simulink model "power_PVarray_3500W"  (R2024b)
settings: Solver=FixedStepDiscrete  StartTime=0.0  StopTime=1.2  RelTol=1e-3
PreLoadFcn:
  | %
  | Fc=3780;                          % PWM Carrier frequency (Hz)
  | Ts_Power=1/Fc/200;         % Simscape Power Systems sample time (s)
  | Ts_Control=20*Ts_Power;  % Inverter Control system sample time (s)
InitFcn:
  | %
  | Fc=3780;                          % PWM Carrier frequency (Hz)
  | Ts_Power=1/Fc/200;         % Simscape Power Systems sample time (s)
  | Ts_Control=20*Ts_Power;  % Inverter Control system sample time (s)
libraries: spsSeriesRLCBranchLib x8, spsGroundLib x4, spsVoltageMeasurementLib x3, spsMeanLib x3, spsCurrentMeasurementLib x2, slpidlib x2, spsParallelRLCLoadLib x2, spsLinearTransformerLib x1, spsSeriesRLCLoadLib x1, spsUniversalBridgeLib x1, spsFundamentalPLLDrivenLib x1, spsPLLLib x1
Description:
  | Copyright 2008-2017 The MathWorks, Inc.
settings Model: Creator=MathWorks  LastModifiedBy=Lenovo
settings SolverCC: AlgebraicLoopSolver=TrustRegion
settings DataIOCC: SaveFormat=Structure  SignalLoggingSaveFormat=ModelDataLogs  SaveOutput=off  SignalLogging=off  DSMLogging=off  SaveTime=off  ReturnWorkspaceOutputs=off
settings OptimizationCC: ExpressionDepthLimit=2147483647  LifeSpan=inf
settings DebuggingCC: UnderspecifiedInitializationDetection=Classic  MergeDetectMultiDrivingBlocksExec=none  SolverPrmCheckMsg=warning  FcnCallInpInsideContextMsg=warning  UnconnectedInputMsg=warning  UnconnectedOutputMsg=warning  UnconnectedLineMsg=warning  AllowSymbolicDim=off  StateNameClashWarn=warning  SFUnexpectedBacktrackingDiag=warning  SFNoUnconditionalDefaultTransitionDiag=warning  SFExecutionAtInitializationDiag=none  ArithmeticOperatorsInVariantConditions=warning
settings HardwareCC: ProdBitPerPointer=32  ProdBitPerSizeT=32  ProdBitPerPtrDiffT=32  ProdLargestAtomicFloat=None  ProdIntDivRoundTo=Undefined  ProdEndianess=Unspecified  ProdWordSize=32  ProdHWDeviceType=32-bit Generic
settings ModelReferenceCC: EnableRefExpFcnMdlSchedulingChecks=on  PropagateSignalLabelsOutOfModel=off
settings SFSimCC: SimUseLocalCustomCode=off  CustomCodeUndefinedFunction=UseInterfaceOnly
settings RTWCC: RTWUseLocalCustomCode=off  GPUComputeCapability=3.5
settings CodeAppCC: StateflowObjectComments=on
settings GRTTargetCC: TargetLangStandard=C89/C90 (ANSI)  CombineOutputUpdateFcns=off  GRTInterface=on
settings ConfigComp: CovMetricSettings=dw  CovSaveCumulativeToWorkspaceVar=on  CovSaveSingleToWorkspaceVar=on  CovExternalEMLEnable=off  CovSFcnEnable=off
settings SimscapeCC: SimscapeNormalizeSystem=off

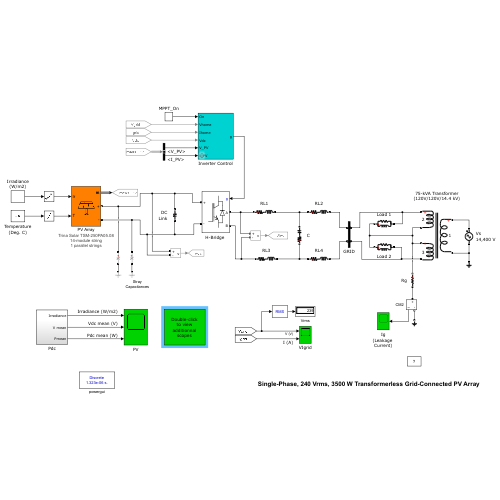
[thumbnail: Simulink's stored preview of the top-level diagram]
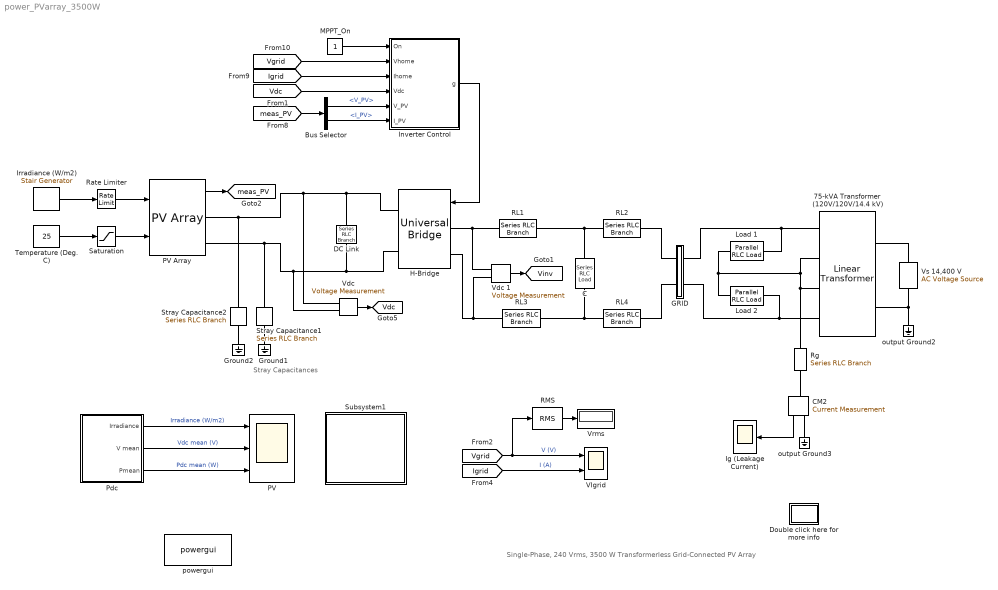
== system power_PVarray_3500W ==
  note: Single-Phase, 240 Vrms, 3500 W Transformerless Grid-Connected PV Array
  note: Stray
      | Capacitances
  75-kVA Transformer (120V/120V/14.4 kV) : spsLinearTransformerLib/Linear Transformer  UNITS=pu  NominalPower=[75e3,60]  winding1=[14.4e3 0.01,0.03]  winding2=[120,0.02,0]  ThreeWindings=on  winding3=[120,0.02,0]  RmLm=[50,50]  Measurements=None  DataType=off
  Bus Selector : BusSelector  OutputSignals=V_PV,I_PV
  C : spsSeriesRLCLoadLib/Series RLC Load  LConnTagsString=a  RConnTagsString=__new0  NominalVoltage=240  NominalFrequency=60  ActivePower=10.5  InductivePower=0  CapacitivePower=525  Setx0=off  InitialVoltage=0  SetiL0=off  InitialCurrent=0  Measurements=None  LoadType=constant Z
  CM2 : spsCurrentMeasurementLib/Current Measurement  PhasorSimulation=off  OutputType=Complex  PSBequivalent=0
  DC Link : spsSeriesRLCBranchLib/Series RLC Branch  LConnTagsString=__new0  RConnTagsString=__new0  BranchType=C  Resistance=1.0  Inductance=1.0  SetiL0=off  InitialCurrent=0  Capacitance=3000e-6  Setx0=on  InitialVoltage=425  Measurements=None
  Double click here for more info : Subsystem
      settings: OpenFcn=showdemo(bdroot(gcb))
      mask Display: disp('?')
  GRID : Subsystem
  Ground1 : spsGroundLib/Ground  LConnTagsString=a
  Ground2 : spsGroundLib/Ground  LConnTagsString=a
  "H-Bridge " : spsUniversalBridgeLib/Universal Bridge  Arms=2  SnubberResistance=1e6  SnubberCapacitance=inf  Device=IGBT / Diodes  Ron=1e-3  Lon=0  ForwardVoltages=[ 0 0 ]  ForwardVoltage=0  GTOparameters=[ 10e-6 , 20e-6 ]  IGBTparameters=[ 1e-6 , 2e-6 ]*0  Measurements=None  Measurements_2=None  converterType=Rectifier
  Ig (Leakage Current) : Scope
  Inverter Control : Subsystem  mask(Inverter Control){Pnom=3500, Fnom=60, Vnom_prim=240, Vnom_dc=400, Increment_MPPT=0.003, Limits_MPPT=[ 450 375 ], Vdc_ref_Init=425, Kp_VDCreg=12, Ki_VDCreg=200, Kp_Ireg=0.15, Ki_Ireg=6.6, RLff=[ 0.002 0.20 ], Fc=3780, PWMmode12=Bipolar, Ts_Control=Ts_Control, Ts_PWMgenerator=Ts_Power}
      mask prompts: Pnom "Power (VA)"; Fnom "Frequency (Hz)"; Vnom_prim "Primary voltage (Vrms LL)"; Vnom_dc "DC voltage (V)"; Increment_MPPT "Output increment (V)"; Limits_MPPT "Output limits [ Upper  Lower ]"; Vdc_ref_Init "Output initial value (V)"; Kp_VDCreg "Proportional gain"; Ki_VDCreg "Integral gain"; Kp_Ireg "Proportional gain"; Ki_Ireg "Integral gain"; RLff "Feedforward Values [Rff Lff] (pu)"; Fc "Carrier frequency (Hz)"; PWMmode12 "PWM method"; Ts_Control "Control systems"; Ts_PWMgenerator "PWM generator"
      mask help:
      | The main components of the Inverter Control are:
      | 1. PLL & Measurements
      | 2. Maximum Power Point Tracker System (MPPT) using a Perturb & Observe algorithm
      | 3. DC Voltage Regulator
      | 4. Current Regulator
      | 5. PWM Modulator
      mask init:
      | blockName=gcb;
      | if PWMmode12==1
      |     set_param([blockName,'/','PWM_Generator'],'ModulatorType','Single-phase full-bridge (4 pulses)')
      | else
      |     set_param([blockName,'/','PWM_Generator'],'ModulatorType','Single-phase full-bridge - Bipolar modulation (4 pulses)')
      | end
      mask TypeOptions PWMmode12: Unipolar | Bipolar
      mask DialogControl Container4 Prompt: Nominal Values:
      mask DialogControl Container3 Prompt: MPPT Controller:
      mask DialogControl Container8 Prompt: Dc Voltage Regulator:
      mask DialogControl Container6 Prompt: Current Regulator:
      mask DialogControl Container9 Prompt: PWM Modulator:
      mask DialogControl SampleTimes Prompt: Sample Times:
  Irradiance (W/m2) : spsStairGeneratorLib/Stair Generator  t=[0, 0.4]  e=[0.25, 0.75]*1000  Ts=Ts_Power
  Load 1 : spsParallelRLCLoadLib/Parallel RLC Load  LConnTagsString=a  RConnTagsString=__new0  NominalVoltage=120  NominalFrequency=60  ActivePower=5e3  InductivePower=2e3  CapacitivePower=0  Setx0=off  InitialVoltage=0  SetiL0=off  InitialCurrent=0  Measurements=None  LoadType=constant Z
      settings: AttributesFormatString=\n  LibrarySourceBlock=sps_lib/Passives/Parallel RLC Load
  Load 2 : spsParallelRLCLoadLib/Parallel RLC Load  LConnTagsString=a  RConnTagsString=__new0  NominalVoltage=120  NominalFrequency=60  ActivePower=5e3  InductivePower=2e3  CapacitivePower=0  Setx0=off  InitialVoltage=0  SetiL0=off  InitialCurrent=0  Measurements=None  LoadType=constant Z
      settings: AttributesFormatString=\n  LibrarySourceBlock=sps_lib/Passives/Parallel RLC Load
  MPPT_On : Constant
  PV : Scope  NumInputPorts=3
  PV Array : spsPVArrayLib/PV Array  Npar=1  Nser=14  PlotType=array @ 1000 W/m2 & specified temperatures  S_vec="[ 1000  500  100 ]"  Temp_C_vec=[ 45 25 100 ]  ModuleName=Trina Solar TSM-250PA05.08  PlotWhenSelected=off  Pm=249.86  Ncell=60  Voc=37.6  Isc=8.55  Vm=31  Im=8.06  beta_Voc_pc=-0.35  alpha_Isc_pc=0.06  beta_Voc=-0.1316  alpha_Isc=0.00513  IL=8.5795  I0=2.0381e-10  nI=0.99766  Rsh=301.8149  Rs=0.247  RobustModel=off  RobustCellTemperature=313.3991  BAL=on  Tc=1e-6  Tfilter=5e-5
      settings: AttributesFormatString=|
      | %<ModuleName>
      | %<Nser>-module string
      | %<Npar> parallel strings
  Pdc : Subsystem
  RL{1..4} (4 alike) : spsSeriesRLCBranchLib/Series RLC Branch  LConnTagsString=__new0  RConnTagsString=__new0  BranchType=RL  Resistance=8.23e-3  Inductance=2.183e-3  SetiL0=off  InitialCurrent=0  Capacitance=1e-6  Setx0=off  InitialVoltage=0  Measurements=None
  RMS : spsRMSLib/RMS  TrueRMS=on  Freq=60  RMSInit=240  Ts=Ts_Power
  Rate Limiter : RateLimiter  RisingSlewLimit=8000  FallingSlewLimit=-8000  SampleTimeMode=inherited  InitialCondition=1000
  Rg : spsSeriesRLCBranchLib/Series RLC Branch  LConnTagsString=__new0  RConnTagsString=__new0  BranchType=R  Resistance=0.2  Inductance=1  SetiL0=off  InitialCurrent=0  Capacitance=50e-9  Setx0=off  InitialVoltage=0  Measurements=None
  Saturation : Saturate  UpperLimit=55  LowerLimit=5
  Stray Capacitance1 : spsSeriesRLCBranchLib/Series RLC Branch  LConnTagsString=__new0  RConnTagsString=__new0  BranchType=C  Resistance=1e-3  Inductance=1  SetiL0=off  InitialCurrent=0  Capacitance=4e-9  Setx0=off  InitialVoltage=0  Measurements=None
  Stray Capacitance2 : spsSeriesRLCBranchLib/Series RLC Branch  LConnTagsString=__new0  RConnTagsString=__new0  BranchType=C  Resistance=1e-3  Inductance=1  SetiL0=off  InitialCurrent=0  Capacitance=4e-9  Setx0=off  InitialVoltage=0  Measurements=None
  Subsystem1 : Subsystem
      mask Display: disp('Double-click\nto view\nadditionnal\nscopes')
  Temperature (Deg. C) : Constant  Value=25
  VIgrid : Scope  NumInputPorts=2
  "Vdc " : spsVoltageMeasurementLib/Voltage Measurement  Tag=PoWeRsYsTeMmEaSuReMeNt  PhasorSimulation=off  OutputType=Magnitude  PSBequivalent=0
  Vdc 1 : spsVoltageMeasurementLib/Voltage Measurement  Tag=PoWeRsYsTeMmEaSuReMeNt  PhasorSimulation=off  OutputType=Magnitude  PSBequivalent=0
  Vrms : Display
      settings: Decimation=200
  Vs 14,400 V : spsACVoltageSourceLib/AC Voltage Source  Description=source block  Amplitude=14400*sqrt(2)  Phase=0  Frequency=60  SampleTime=0  Measurements=None  BusType=swing  Pref=10e3  Qref=0  Qmin=-inf  Qmax=+inf
      settings: AttributesFormatString=\n
  output Ground2 : spsGroundLib/Ground  LConnTagsString=a
  output Ground3 : spsGroundLib/Ground  LConnTagsString=a
  powergui : sps_lib/powergui  Priority=1  SimulationMode=Discrete  SampleTime=Ts_Power  frequency=60  Iterations=50  frequencyindice=0  Pbase=100e6  ErrMax=1e-4  UnitsV=kV  UnitsW=MW  buscounter=0  FunctionMessages=off  echomessages=off  EnableUseOfTLC=off  CurrentSourceSwitches=off  DisableSnubberDevices=off  DisableRonSwitches=off  DisableVfSwitches=off  DisplayEquations=off  AutomaticDiscreteSolvers=off  SolverType=Tustin/Backward Euler (TBE)  Interpol=off  ExternalGateDelay=off  methode=off  Ts=0  x0status=blocks  SPID=off  SwTol=0  HookPort=off  NonlinearTolerance=1e-4  nMaxIteration=100  ContinueOnMaxIteration=off  RestoreLinks=warning  ResistiveCurrentMeasurement=off  Frange=[0:2:500]  Ylog=off  Xlog=on  ShowGrid=off  save=off  variable=ZData  structure=VIgrid  ZoomFFT=off  StartTime=0.55  cycles=1  DisplayStyle=1  fundamental=60  FreqAxis=on  MaxFrequency=10000  frequencyindicesteady=1  RmsSteady=1  display=off
  tag scope: Vdc=global, Vinv=global, meas_PV=global
  wires:
  Vdc 1/1 -> [Vinv]
  [Igrid] -> VIgrid/2  "I (A)"
  Irradiance (W/m2)/1 -> Rate Limiter/1
  Temperature (Deg. C)/1 -> Saturation/1
  Rate Limiter/1 -> PV Array/1
  Saturation/1 -> PV Array/2
  PV Array/1 -> [meas_PV]
  [Vgrid] -> Inverter Control/2(Vhome)
  [Igrid] -> Inverter Control/3(Ihome)
  [Vdc] -> Inverter Control/4(Vdc)
  [meas_PV] -> Bus Selector/1
  "Vdc "/1 -> [Vdc]
  Bus Selector/1 -> Inverter Control/5(V_PV)  "<V_PV>"
  Bus Selector/2 -> Inverter Control/6(I_PV)  "<I_PV>"
  MPPT_On/1 -> Inverter Control/1(On)
  Pdc/2(V mean) -> PV/2  "Vdc mean (V)"
  Pdc/3(Pmean) -> PV/3  "Pdc mean (W)"
  Inverter Control/1(g) -> "H-Bridge "/1
  CM2/1 -> Ig (Leakage Current)/1
  Pdc/1(Irradiance) -> PV/1  "Irradiance (W/m2)"
  [Vgrid] -> VIgrid/1, RMS/1  "V (V)"
  RMS/1 -> Vrms/1
  connections:
  PV Array/RConn1 -- Stray Capacitance2/LConn1 -- "Vdc "/LConn1 -- "H-Bridge "/RConn1 -- DC Link/LConn1
  "H-Bridge "/LConn1 -- Vdc 1/LConn1 -- RL1/LConn1
  "H-Bridge "/LConn2 -- RL3/LConn1 -- Vdc 1/LConn2
  RL1/RConn1 -- RL2/LConn1 -- C/RConn1
  C/LConn1 -- RL3/RConn1 -- RL4/LConn1
  "H-Bridge "/RConn2 -- Stray Capacitance1/LConn1 -- PV Array/RConn2 -- "Vdc "/LConn2 -- DC Link/RConn1
  RL2/RConn1 -- GRID/LConn1
  RL4/RConn1 -- GRID/LConn2
  output Ground2/LConn1 -- Vs 14,400 V/LConn1 -- 75-kVA Transformer (120V/120V/14.4 kV)/LConn2
  Vs 14,400 V/RConn1 -- 75-kVA Transformer (120V/120V/14.4 kV)/LConn1
  Load 2/RConn1 -- GRID/RConn2 -- 75-kVA Transformer (120V/120V/14.4 kV)/RConn4
  Load 1/RConn1 -- GRID/RConn1 -- 75-kVA Transformer (120V/120V/14.4 kV)/RConn1
  Load 1/LConn1 -- 75-kVA Transformer (120V/120V/14.4 kV)/RConn2 -- Rg/LConn1 -- 75-kVA Transformer (120V/120V/14.4 kV)/RConn3 -- Load 2/LConn1
  Ground1/LConn1 -- Stray Capacitance1/RConn1
  Ground2/LConn1 -- Stray Capacitance2/RConn1
  CM2/LConn1 -- Rg/RConn1
  CM2/RConn1 -- output Ground3/LConn1

== system power_PVarray_3500W/Double click here for more info ==

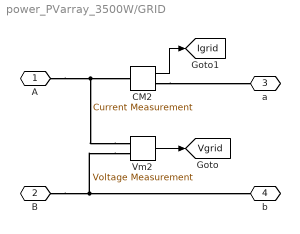
== system power_PVarray_3500W/GRID ==
  CM2 : spsCurrentMeasurementLib/Current Measurement  PhasorSimulation=off  OutputType=Complex  PSBequivalent=0
  Vm2 : spsVoltageMeasurementLib/Voltage Measurement  PhasorSimulation=off  OutputType=Complex  PSBequivalent=0
  A : PMIOPort  Side=Left
  B : PMIOPort  Port=2  Side=Left
  a : PMIOPort  Port=3  Side=Right
  b : PMIOPort  Port=4  Side=Right
  tag scope: Igrid=global, Vgrid=global
  wires:
  Vm2/1 -> [Vgrid]
  CM2/1 -> [Igrid]
  connections:
  Vm2/LConn2 -- b/RConn1 -- B/RConn1
  Vm2/LConn1 -- A/RConn1 -- CM2/LConn1
  CM2/RConn1 -- a/RConn1

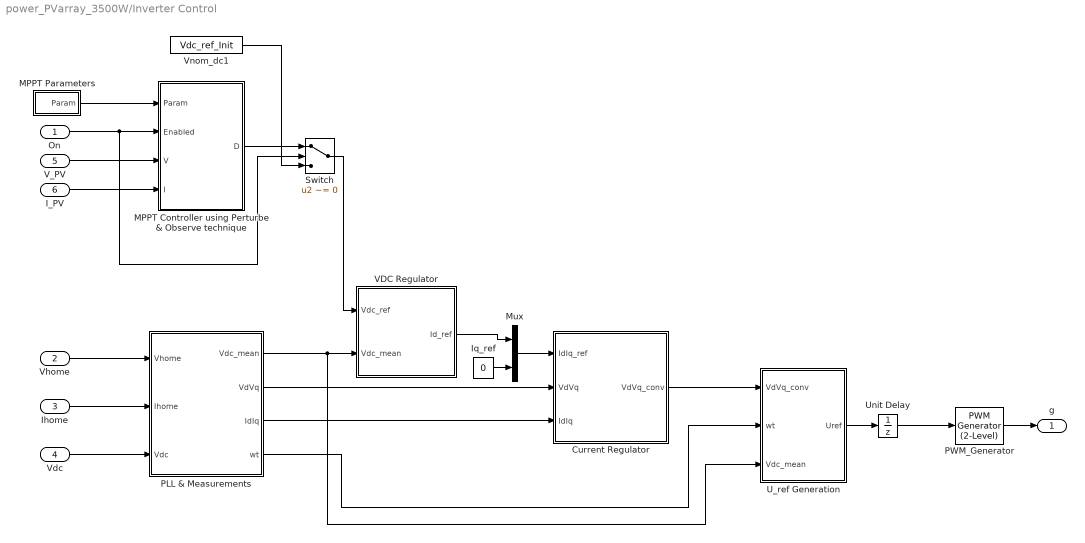
== system power_PVarray_3500W/Inverter Control ==
  On : Inport  PortDimensions=1
  Vhome : Inport  Port=2  PortDimensions=1
  Ihome : Inport  Port=3  PortDimensions=1
  Vdc : Inport  Port=4  PortDimensions=1
  V_PV : Inport  Port=5  PortDimensions=1
  I_PV : Inport  Port=6  PortDimensions=1
  Current Regulator : Subsystem
  Iq_ref : Constant  Value=0
  MPPT Parameters : Subsystem
  "MPPT Controller using Perturbe & Observe technique " : MATLAB Function  TreatAsAtomicUnit=on
  Mux : Mux  Inputs=2
  PLL & Measurements : Subsystem
  PWM_Generator : spsPWMGenerator2LevelLib/PWM Generator (2-Level)  ModulatorType=Single-phase full-bridge - Bipolar modulation (4 pulses)  ModulatorMode=Unsynchronized  Fc=Fc  Pc=90  nF=27  MinMax="[ -1  1 ]"  SamplingTechnique=Asymmetrical regular (double edge)  ModulatingSignals=off  m=0.8  Freq=60  Phase=0  Ts=Ts_PWMgenerator  ShowCarrierOutport=off
      settings: AttributesFormatString=%<ModulatorType>
  Switch : Switch  Criteria=u2 ~= 0  SaturateOnIntegerOverflow=off  InputSameDT=off
  "U_ref Generation " : Subsystem
  Unit Delay : UnitDelay  InitialCondition=0.1684  SampleTime=Ts_Control  HasFrameUpgradeWarning=on
  VDC Regulator : Subsystem
  Vnom_dc1 : Constant  Value=Vdc_ref_Init
  g : Outport  VectorParamsAs1DForOutWhenUnconnected=off
  wires:
  Iq_ref/1 -> Mux/2
  Vhome/1 -> PLL & Measurements/1(Vhome)
  Ihome/1 -> PLL & Measurements/2(Ihome)
  V_PV/1 -> "MPPT Controller using Perturbe & Observe technique "/3(V)
  I_PV/1 -> "MPPT Controller using Perturbe & Observe technique "/4(I)
  MPPT Parameters/1(Param) -> "MPPT Controller using Perturbe & Observe technique "/1(Param)
  On/1 -> "MPPT Controller using Perturbe & Observe technique "/2(Enabled), Switch/2
  Unit Delay/1 -> PWM_Generator/1
  "MPPT Controller using Perturbe & Observe technique "/1(D) -> Switch/1
  Vdc/1 -> PLL & Measurements/3(Vdc)
  Vnom_dc1/1 -> Switch/3
  PLL & Measurements/2(VdVq) -> Current Regulator/2(VdVq)
  PLL & Measurements/3(IdIq) -> Current Regulator/3(IdIq)
  Mux/1 -> Current Regulator/1(IdIq_ref)
  VDC Regulator/1(Id_ref) -> Mux/1
  PLL & Measurements/1(Vdc_mean) -> "U_ref Generation "/3(Vdc_mean), VDC Regulator/2(Vdc_mean)
  Current Regulator/1(VdVq_conv) -> "U_ref Generation "/1(VdVq_conv)
  PLL & Measurements/4(wt) -> "U_ref Generation "/2(wt)
  "U_ref Generation "/1(Uref) -> Unit Delay/1
  PWM_Generator/1 -> g/1
  Switch/1 -> VDC Regulator/1(Vdc_ref)

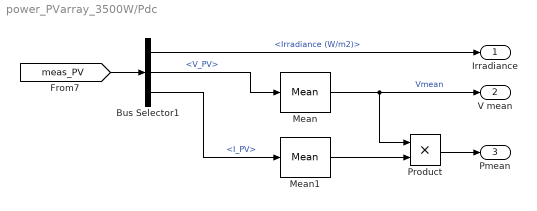
== system power_PVarray_3500W/Pdc ==
  Bus Selector1 : BusSelector  OutputSignals=Irradiance (W/m2),V_PV,I_PV
  Mean : spsMeanLib/Mean  Freq=60  Vinit=406  Ts=Ts_Control
  Mean1 : spsMeanLib/Mean  Freq=60  Vinit=8.05  Ts=Ts_Control
  Product : Product
  Irradiance : Outport  VectorParamsAs1DForOutWhenUnconnected=off
  V mean : Outport  Port=2  VectorParamsAs1DForOutWhenUnconnected=off
  Pmean : Outport  Port=3  VectorParamsAs1DForOutWhenUnconnected=off
  wires:
  Mean/1 -> Product/1, V mean/1  "Vmean"
  Mean1/1 -> Product/2
  Product/1 -> Pmean/1
  [meas_PV] -> Bus Selector1/1
  Bus Selector1/2 -> Mean/1  "<V_PV>"
  Bus Selector1/3 -> Mean1/1  "<I_PV>"
  Bus Selector1/1 -> Irradiance/1  "<Irradiance (W/m2)>"

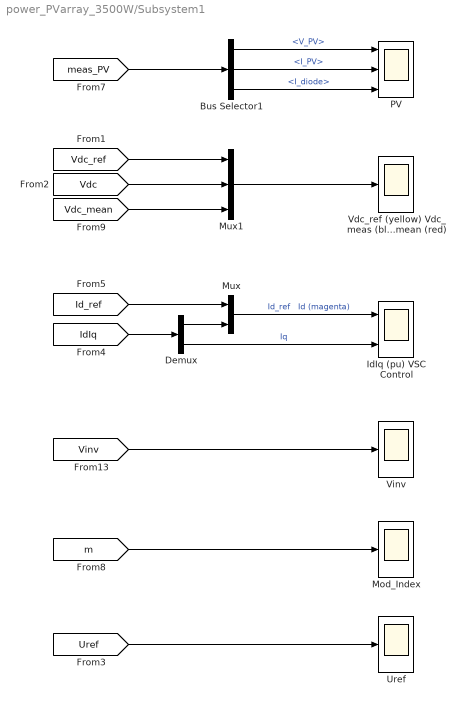
== system power_PVarray_3500W/Subsystem1 ==
  Bus Selector1 : BusSelector  OutputSignals=V_PV,I_PV,I_diode
  Demux : Demux  Outputs=2
  IdIq (pu) VSC Control : Scope  NumInputPorts=2
  Mod_Index : Scope
  Mux : Mux  Inputs=2
  Mux1 : Mux  Inputs=3
  PV : Scope  NumInputPorts=3
  Uref : Scope
  Vdc_ref (yellow) Vdc_meas (blue) Vdc_mean (red) : Scope
  Vinv : Scope
  wires:
  [m] -> Mod_Index/1
  Bus Selector1/2 -> PV/2  "<I_PV>"
  Bus Selector1/1 -> PV/1  "<V_PV>"
  Bus Selector1/3 -> PV/3  "<I_diode>"
  [meas_PV] -> Bus Selector1/1
  [Vdc] -> Mux1/2
  [Vdc_ref] -> Mux1/1
  Demux/2 -> IdIq (pu) VSC Control/2  "Iq"
  Mux/1 -> IdIq (pu) VSC Control/1  "Id_ref   Id (magenta)"
  Demux/1 -> Mux/2
  [Id_ref] -> Mux/1
  [IdIq] -> Demux/1
  [Vdc_mean] -> Mux1/3
  [Vinv] -> Vinv/1
  [Uref] -> Uref/1
  Mux1/1 -> Vdc_ref (yellow) Vdc_meas (blue) Vdc_mean (red)/1

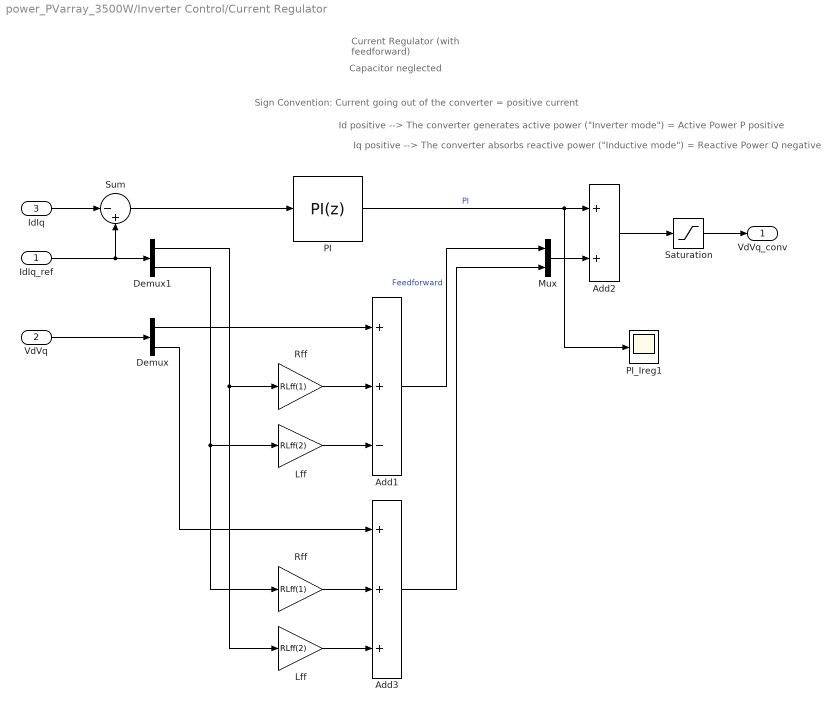
== system power_PVarray_3500W/Inverter Control/Current Regulator ==
  note: Id positive --> The converter generates active power ("Inverter mode") = Active Power P positive
  note: Iq positive --> The converter absorbs reactive power ("Inductive mode") = Reactive Power Q negative
  note: Sign Convention: Current going out of the converter = positive current
  note: Current Regulator
      | (with feedforward)
  note: Capacitor neglected
  IdIq_ref : Inport  PortDimensions=2
  VdVq : Inport  Port=2  PortDimensions=2
  IdIq : Inport  Port=3  PortDimensions=2
  Add1 : Sum  Inputs=++-
  Add2 : Sum
  Add3 : Sum  Inputs=+++
  Demux : Demux  Outputs=2
  Demux1 : Demux  Outputs=2
  Lff : Gain  Gain=RLff(2)  SaturateOnIntegerOverflow=on  OutDataTypeStr=Inherit: Same as input  ParamDataTypeStr=Inherit: Same as input
  "Lff  " : Gain  Gain=RLff(2)  SaturateOnIntegerOverflow=on  OutDataTypeStr=Inherit: Same as input  ParamDataTypeStr=Inherit: Same as input
  Mux : Mux  Inputs=2
  PI : slpidlib/PID Controller  Controller=PI  Form=Parallel  TimeDomain=Discrete-time  UseExternalTs=off  SampleTime=Ts_Control  IntegratorMethod=Forward Euler  FilterMethod=Forward Euler  ControllerParametersSource=internal  P=Kp_Ireg  I=Ki_Ireg  UseKiTs=off  D=0  UseExternalDerivativeSource=off  N=100  UseFilter=on  TunerSelectOption=Transfer Function Based (PID Tuner App)  InitialConditionSource=internal  InitialConditionForIntegrator=0  InitialConditionForFilter=0  DifferentiatorICPrevScaledInput=0  ExternalReset=none  TrackingMode=off  Kt=1  LimitOutput=on  SatLimitsSource=internal  UpperSaturationLimit=1.5  LowerSaturationLimit=-1.5  LinearizeAsGain=off  AntiWindupMode=none  Kb=1  LimitIntegrator=off  UpperIntegratorSaturationLimit=inf  LowerIntegratorSaturationLimit=-inf  POutMin=[]  POutMax=[]  IOutMin=[]  IOutMax=[]  DOutMin=[]  DOutMax=[]  NOutMin=[]  NOutMax=[]  SumOutMin=[]  SumOutMax=[]  SaturationOutMin=[]  SaturationOutMax=[]  PParamMin=[]  PParamMax=[]  IParamMin=[]  IParamMax=[]  DParamMin=[]  DParamMax=[]  NParamMin=[]  NParamMax=[]  KbParamMin=[]  KbParamMax=[]  KtParamMin=[]  KtParamMax=[]  KbOutMin=[]  KbOutMax=[]  KtOutMin=[]  KtOutMax=[]  IntegratorOutMin=[]  IntegratorOutMax=[]  FilterOutMin=[]  FilterOutMax=[]  SumI1OutMin=[]  SumI1OutMax=[]  SumI2OutMin=[]  SumI2OutMax=[]  SumI3OutMin=[]  SumI3OutMax=[]  SumI4OutMin=[]  SumI4OutMax=[]  SumDOutMin=[]  SumDOutMax=[]  DifferentiatorOutMin=[]  DifferentiatorOutMax=[]  FilterDiffOutCoefMin=[]  FilterDiffOutCoefMax=[]  ReciprocalOutMin=[]  ReciprocalOutMax=[]  SumDenOutMin=[]  SumDenOutMax=[]  SumNumOutMin=[]  SumNumOutMax=[]  DivideOutMin=[]  DivideOutMax=[]  UdiffTsProdOutMin=[]  UdiffTsProdOutMax=[]  NTsProdOutMin=[]  NTsProdOutMax=[]  UintegralTsProdOutMin=[]  UintegralTsProdOutMax=[]  UngainTsProdOutMin=[]  UngainTsProdOutMax=[]  ClampingZeroOutDataTypeStr=Inherit: Inherit via back propagation  ClampingZeroOutMin=[]  ClampingZeroOutMax=[]  FilterDenConstantOutDataTypeStr=Inherit: Inherit via back propagation  FilterDenConstantOutMin=[]  FilterDenConstantOutMax=[]  PCopyOutDataTypeStr=Inherit: Inherit via back propagation  PCopyOutMin=[]  PCopyOutMax=[]  NCopyOutDataTypeStr=Inherit: Inherit via back propagation  NCopyOutMin=[]  NCopyOutMax=[]  IntegratorContinuousStateAttributes=''  IntegratorStateMustResolveToSignalObject=off  IntegratorRTWStateStorageClass=Auto  FilterContinuousStateAttributes=''  FilterStateMustResolveToSignalObject=off  FilterRTWStateStorageClass=Auto  ParallelPVariant=InternalParameters  IdealPVariant=Disabled  IVariant=InternalParameters  DVariant=Disabled  IntegratorVariant=Discrete  SatVariant=Enabled  AWVariant=Passthrough  PCopyVariant=Disabled  TRVariant=Disabled  FdbkBlocksVariant=Forward  IdealPFdbkVariant=Disabled  SatFdbkVariant=Disabled  DerivativeFilterVariant=Disabled  NVariant=Disabled  NCopyVariant=Disabled_SignalSpec  FilterICVariant=Disabled  IntegratorICVariant=InternalICs  ExternalResetVariant=Disabled  TRSumVariant=Passthrough  SumFdbkVariant=Disabled  SumVariant=Sum_PI  TsampFilterVariant=InternalTs  TsampNgainVariant=Passthrough  TsampIntegralVariant=Disabled_SignalSpec  ExternalSaturationOutDataTypeStr=Inherit: Same as second input  DerivativeSourceVariant=Disabled  PreIntVariant=InternalPreInt
  PI_Ireg1 : Scope
  Rff : Gain  Gain=RLff(1)  SaturateOnIntegerOverflow=on  OutDataTypeStr=Inherit: Same as input  ParamDataTypeStr=Inherit: Same as input
  "Rff " : Gain  Gain=RLff(1)  SaturateOnIntegerOverflow=on  OutDataTypeStr=Inherit: Same as input  ParamDataTypeStr=Inherit: Same as input
  Saturation : Saturate  UpperLimit=1.5  LowerLimit=-1.5
  Sum : Sum  Inputs=|-+
  VdVq_conv : Outport  VectorParamsAs1DForOutWhenUnconnected=off
  wires:
  Add3/1 -> Mux/2
  Demux/2 -> Add3/1
  Add1/1 -> Mux/1  "Feedforward"
  Lff/1 -> Add3/3
  Rff/1 -> Add3/2
  Demux1/2 -> Rff/1, "Lff  "/1
  "Lff  "/1 -> Add1/3
  Demux1/1 -> Lff/1, "Rff "/1
  "Rff "/1 -> Add1/2
  Demux/1 -> Add1/1
  VdVq/1 -> Demux/1
  Saturation/1 -> VdVq_conv/1
  Add2/1 -> Saturation/1
  IdIq/1 -> Sum/1
  IdIq_ref/1 -> Demux1/1, Sum/2
  Sum/1 -> PI/1
  PI/1 -> Add2/1, PI_Ireg1/1  "PI"
  Mux/1 -> Add2/2

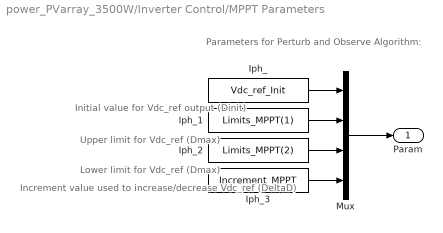
== system power_PVarray_3500W/Inverter Control/MPPT Parameters ==
  note: Upper limit for Vdc_ref (Dmax)
  note: Increment value used to increase/decrease Vdc_ref (DeltaD)
  note: Initial value for Vdc_ref output (Dinit)
  note: Lower limit for Vdc_ref (Dmax)
  note: Parameters for Perturb and Observe Algorithm:
  Iph_ : Constant  Value=Vdc_ref_Init
  Iph_1 : Constant  Value=Limits_MPPT(1)
  Iph_2 : Constant  Value=Limits_MPPT(2)
  Iph_3 : Constant  Value=Increment_MPPT
  Mux : Mux
  Param : Outport  VectorParamsAs1DForOutWhenUnconnected=off
  wires:
  Iph_/1 -> Mux/1
  Iph_1/1 -> Mux/2
  Iph_2/1 -> Mux/3
  Iph_3/1 -> Mux/4
  Mux/1 -> Param/1

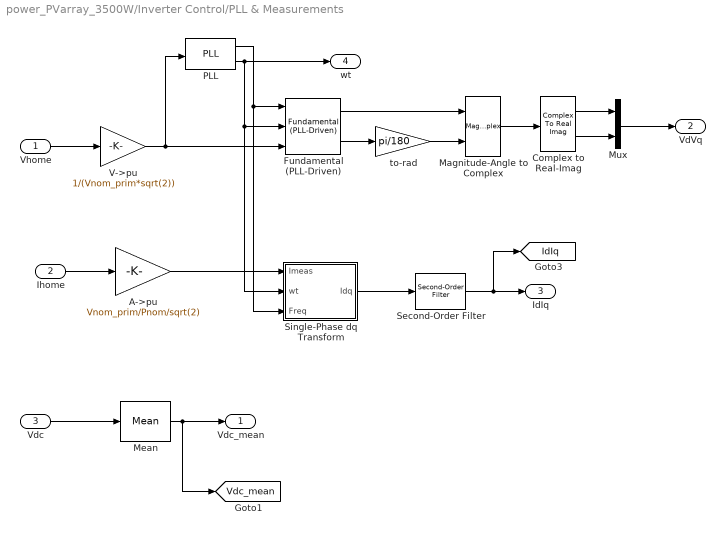
== system power_PVarray_3500W/Inverter Control/PLL & Measurements ==
  Vhome : Inport
  Ihome : Inport  Port=2
  Vdc : Inport  Port=3
  A->pu : Gain  Gain=Vnom_prim/Pnom/sqrt(2)  SaturateOnIntegerOverflow=on  OutDataTypeStr=Inherit: Same as input  ParamDataTypeStr=Inherit: Same as input
  Complex to Real-Imag : ComplexToRealImag
  Fundamental (PLL-Driven) : spsFundamentalPLLDrivenLib/Fundamental (PLL-Driven)  Finit=Fnom  Fmin=45  InInit=[1, 0]  Ts=Ts_Control
      settings: LibrarySourceBlock=|
      | sps_lib/Sensors and Measurements/Fundamental
      | (PLL-Driven)
  Magnitude-Angle to Complex : MagnitudeAngleToComplex
  Mean : spsMeanLib/Mean  Freq=Fnom  Vinit=Vdc_ref_Init  Ts=Ts_Control
  Mux : Mux  Inputs=2
  PLL : spsPLLLib/PLL  Fmin=45  Par_Init=[0, Fnom]  ParK=[180, 3200, 1]  TcD=1e-4  MaxRateChangeFreq=12  FilterCutOffFreq=25  Ts=Ts_Control  AGC=on
      settings: LibrarySourceBlock=sps_lib/Control/PLL
  Second-Order Filter : spsSecondOrderFilterLib/Second-Order Filter  FilterType=Lowpass  Fo=2000  Zeta=1  Ts=Ts_Control  Initialize=on  Vac_Init="[0,  0,  60;0,0,60]"  Vdc_Init=[0.9 0]  PlotResponse=off  FreqRange=[0, 500, 1]
      settings: LibrarySourceBlock=|
      | sps_lib/Control/Filters/Second-Order
      | Filter
  Single-Phase dq Transform : Subsystem
  V->pu : Gain  Gain=1/(Vnom_prim*sqrt(2))  SaturateOnIntegerOverflow=on  OutDataTypeStr=Inherit: Same as input  ParamDataTypeStr=Inherit: Same as input
  to-rad : Gain  Gain=pi/180
  Vdc_mean : Outport  VectorParamsAs1DForOutWhenUnconnected=off
  VdVq : Outport  Port=2  VectorParamsAs1DForOutWhenUnconnected=off
  IdIq : Outport  Port=3  VectorParamsAs1DForOutWhenUnconnected=off
  wt : Outport  Port=4  VectorParamsAs1DForOutWhenUnconnected=off
  tag scope: IdIq=global, Vdc_mean=global
  wires:
  Mean/1 -> Vdc_mean/1, [Vdc_mean]
  Vdc/1 -> Mean/1
  to-rad/1 -> Magnitude-Angle to Complex/2
  Mux/1 -> VdVq/1
  Complex to Real-Imag/2 -> Mux/2
  Complex to Real-Imag/1 -> Mux/1
  Magnitude-Angle to Complex/1 -> Complex to Real-Imag/1
  Fundamental (PLL-Driven)/2 -> to-rad/1
  Fundamental (PLL-Driven)/1 -> Magnitude-Angle to Complex/1
  A->pu/1 -> Single-Phase dq Transform/1(Imeas)
  PLL/1 -> Single-Phase dq Transform/3(Freq), Fundamental (PLL-Driven)/1
  PLL/2 -> wt/1, Fundamental (PLL-Driven)/2, Single-Phase dq Transform/2(wt)
  Ihome/1 -> A->pu/1
  Vhome/1 -> V->pu/1
  V->pu/1 -> Fundamental (PLL-Driven)/3, PLL/1
  Single-Phase dq Transform/1(Idq) -> Second-Order Filter/1
  Second-Order Filter/1 -> [IdIq], IdIq/1

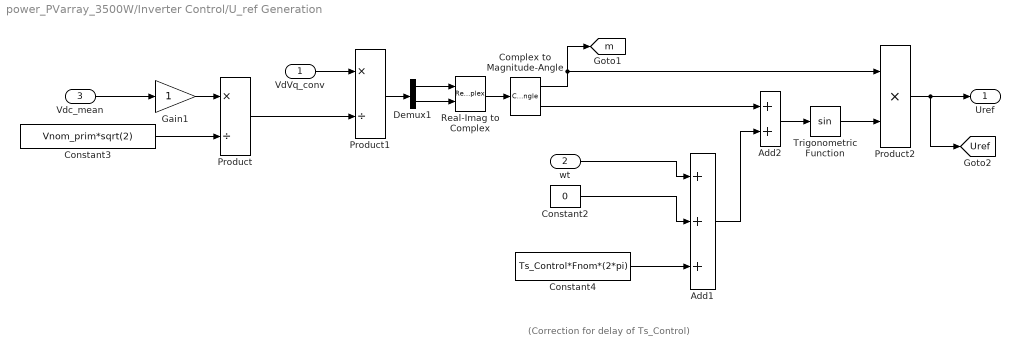
== system power_PVarray_3500W/Inverter Control/U_ref Generation  ==
  note: (Correction for delay of Ts_Control)
  VdVq_conv : Inport
  wt : Inport  Port=2
  Vdc_mean : Inport  Port=3
  Add1 : Sum  Inputs=+++
  Add2 : Sum
  Complex to Magnitude-Angle : ComplexToMagnitudeAngle
  Constant2 : Constant  Value=0
  Constant3 : Constant  Value=Vnom_prim*sqrt(2)
  Constant4 : Constant  Value=Ts_Control*Fnom*(2*pi)
  Demux1 : Demux  Outputs=2
  Gain1 : Gain
  Product : Product  Inputs=*/  RndMeth=Zero
  Product1 : Product  Inputs=*/  RndMeth=Zero
  Product2 : Product  Inputs=**  RndMeth=Zero
  Real-Imag to Complex : RealImagToComplex
  Trigonometric Function : Trigonometry
  Uref : Outport  VectorParamsAs1DForOutWhenUnconnected=off
  tag scope: Uref=global, m=global
  wires:
  VdVq_conv/1 -> Product1/1
  Product2/1 -> Uref/1, [Uref]
  Vdc_mean/1 -> Gain1/1
  Constant4/1 -> Add1/3
  wt/1 -> Add1/1
  Trigonometric Function/1 -> Product2/2
  Complex to Magnitude-Angle/1 -> [m], Product2/1
  Add2/1 -> Trigonometric Function/1
  Add1/1 -> Add2/2
  Complex to Magnitude-Angle/2 -> Add2/1
  Product/1 -> Product1/2
  Constant3/1 -> Product/2
  Constant2/1 -> Add1/2
  Demux1/2 -> Real-Imag to Complex/2
  Demux1/1 -> Real-Imag to Complex/1
  Real-Imag to Complex/1 -> Complex to Magnitude-Angle/1
  Gain1/1 -> Product/1
  Product1/1 -> Demux1/1

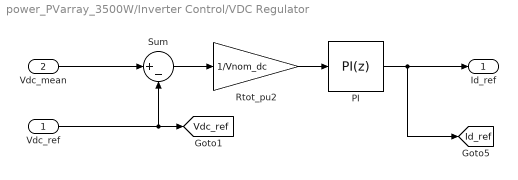
== system power_PVarray_3500W/Inverter Control/VDC Regulator ==
  Vdc_ref : Inport  PortDimensions=1
  Vdc_mean : Inport  Port=2  PortDimensions=1
  PI : slpidlib/PID Controller  Controller=PI  Form=Parallel  TimeDomain=Discrete-time  UseExternalTs=off  SampleTime=Ts_Control  IntegratorMethod=Trapezoidal  FilterMethod=Forward Euler  ControllerParametersSource=internal  P=Kp_VDCreg  I=Ki_VDCreg  UseKiTs=off  D=0  UseExternalDerivativeSource=off  N=100  UseFilter=on  TunerSelectOption=Transfer Function Based (PID Tuner App)  InitialConditionSource=internal  InitialConditionForIntegrator=0.9226  InitialConditionForFilter=0  DifferentiatorICPrevScaledInput=0  ExternalReset=none  TrackingMode=off  Kt=1  LimitOutput=on  SatLimitsSource=internal  UpperSaturationLimit=1.5  LowerSaturationLimit=-1.5  LinearizeAsGain=off  AntiWindupMode=none  Kb=1  LimitIntegrator=off  UpperIntegratorSaturationLimit=inf  LowerIntegratorSaturationLimit=-inf  POutMin=[]  POutMax=[]  IOutMin=[]  IOutMax=[]  DOutMin=[]  DOutMax=[]  NOutMin=[]  NOutMax=[]  SumOutMin=[]  SumOutMax=[]  SaturationOutMin=[]  SaturationOutMax=[]  PParamMin=[]  PParamMax=[]  IParamMin=[]  IParamMax=[]  DParamMin=[]  DParamMax=[]  NParamMin=[]  NParamMax=[]  KbParamMin=[]  KbParamMax=[]  KtParamMin=[]  KtParamMax=[]  KbOutMin=[]  KbOutMax=[]  KtOutMin=[]  KtOutMax=[]  IntegratorOutMin=[]  IntegratorOutMax=[]  FilterOutMin=[]  FilterOutMax=[]  SumI1OutMin=[]  SumI1OutMax=[]  SumI2OutMin=[]  SumI2OutMax=[]  SumI3OutMin=[]  SumI3OutMax=[]  SumI4OutMin=[]  SumI4OutMax=[]  SumDOutMin=[]  SumDOutMax=[]  DifferentiatorOutMin=[]  DifferentiatorOutMax=[]  FilterDiffOutCoefMin=[]  FilterDiffOutCoefMax=[]  ReciprocalOutMin=[]  ReciprocalOutMax=[]  SumDenOutMin=[]  SumDenOutMax=[]  SumNumOutMin=[]  SumNumOutMax=[]  DivideOutMin=[]  DivideOutMax=[]  UdiffTsProdOutMin=[]  UdiffTsProdOutMax=[]  NTsProdOutMin=[]  NTsProdOutMax=[]  UintegralTsProdOutMin=[]  UintegralTsProdOutMax=[]  UngainTsProdOutMin=[]  UngainTsProdOutMax=[]  ClampingZeroOutDataTypeStr=Inherit: Inherit via back propagation  ClampingZeroOutMin=[]  ClampingZeroOutMax=[]  FilterDenConstantOutDataTypeStr=Inherit: Inherit via back propagation  FilterDenConstantOutMin=[]  FilterDenConstantOutMax=[]  PCopyOutDataTypeStr=Inherit: Inherit via back propagation  PCopyOutMin=[]  PCopyOutMax=[]  NCopyOutDataTypeStr=Inherit: Inherit via back propagation  NCopyOutMin=[]  NCopyOutMax=[]  IntegratorContinuousStateAttributes=''  IntegratorStateMustResolveToSignalObject=off  IntegratorRTWStateStorageClass=Auto  FilterContinuousStateAttributes=''  FilterStateMustResolveToSignalObject=off  FilterRTWStateStorageClass=Auto  ParallelPVariant=InternalParameters  IdealPVariant=Disabled  IVariant=InternalParameters  DVariant=Disabled  IntegratorVariant=Discrete  SatVariant=Enabled  AWVariant=Passthrough  PCopyVariant=Disabled  TRVariant=Disabled  FdbkBlocksVariant=Forward  IdealPFdbkVariant=Disabled  SatFdbkVariant=Disabled  DerivativeFilterVariant=Disabled  NVariant=Disabled  NCopyVariant=Disabled_SignalSpec  FilterICVariant=Disabled  IntegratorICVariant=InternalICs  ExternalResetVariant=Disabled  TRSumVariant=Passthrough  SumFdbkVariant=Disabled  SumVariant=Sum_PI  TsampFilterVariant=InternalTs  TsampNgainVariant=Passthrough  TsampIntegralVariant=Disabled_SignalSpec  ExternalSaturationOutDataTypeStr=Inherit: Same as second input  DerivativeSourceVariant=Disabled  PreIntVariant=InternalPreInt
  Rtot_pu2 : Gain  Gain=1/Vnom_dc  SaturateOnIntegerOverflow=on  OutDataTypeStr=Inherit: Same as input  ParamDataTypeStr=Inherit: Same as input
  Sum : Sum  Inputs=|+-
  Id_ref : Outport  InitialOutput=0  VectorParamsAs1DForOutWhenUnconnected=off
  tag scope: Id_ref=global, Vdc_ref=global
  wires:
  Rtot_pu2/1 -> PI/1
  Vdc_ref/1 -> Sum/2, [Vdc_ref]
  Vdc_mean/1 -> Sum/1
  Sum/1 -> Rtot_pu2/1
  PI/1 -> Id_ref/1, [Id_ref]

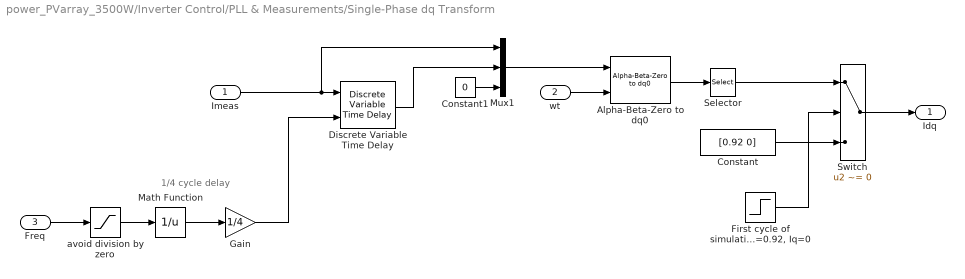
== system power_PVarray_3500W/Inverter Control/PLL & Measurements/Single-Phase dq Transform ==
  note: 1/4 cycle delay
  Imeas : Inport
  wt : Inport  Port=2
  Freq : Inport  Port=3
  Alpha-Beta-Zero to dq0 : spsAlphaBetaZerotodq0Lib/Alpha-Beta-Zero to dq0  Alignment=90 degrees behind phase A axis
  Constant : Constant  Value=[0.92 0]
  Constant1 : Constant  Value=0
  Discrete Variable Time Delay : spsDiscreteVariableTimeDelayLib/Discrete Variable Time Delay  MaxDelay=1  InitialValue=0  Ts=Ts_Control  DFT=on
      settings: LibrarySourceBlock=|
      | sps_lib/Control/Discrete Variable
      | Time Delay
  "First cycle of simulation Id=0.92, Iq=0" : Step  Time=1/Fnom  SampleTime=Ts_Control
  Gain : Gain  Gain=1/4
  Math Function : Math  Operator=reciprocal  SignedPower=on
  Mux1 : Mux  Inputs=3
  Selector : Selector  InputPortWidth=3  IndexOptions=Index vector (dialog)  Indices=[1 2]  OutputSizes=1
  Switch : Switch  Criteria=u2 ~= 0  SaturateOnIntegerOverflow=off  InputSameDT=off
  avoid division by zero : Saturate  UpperLimit=70  LowerLimit=40
  Idq : Outport  VectorParamsAs1DForOutWhenUnconnected=off
  wires:
  Constant1/1 -> Mux1/3
  Discrete Variable Time Delay/1 -> Mux1/2
  Mux1/1 -> Alpha-Beta-Zero to dq0/1
  Imeas/1 -> Discrete Variable Time Delay/1, Mux1/1
  wt/1 -> Alpha-Beta-Zero to dq0/2
  Alpha-Beta-Zero to dq0/1 -> Selector/1
  Freq/1 -> avoid division by zero/1
  avoid division by zero/1 -> Math Function/1
  Math Function/1 -> Gain/1
  Gain/1 -> Discrete Variable Time Delay/2
  Selector/1 -> Switch/1
  Switch/1 -> Idq/1
  Constant/1 -> Switch/3
  "First cycle of simulation Id=0.92, Iq=0"/1 -> Switch/2

== matlab function power_PVarray_3500W/Inverter Control/MPPT Controller using Perturbe & Observe technique  ==
  settings: updateMethod=DISCRETE  sampleTime=Ts_Control
  data: Param input; Enabled input; V input; I input; D output
function D  = PandO(Param, Enabled, V, I)

% MPPT controller based on the Perturb & Observe algorithm.

% D output = Reference for DC link voltage (Vdc_ref) 
%
% Enabled input = 1 to enable the MPPT controller
% V input = PV array terminal voltage (V)
% I input = PV array current (A)
%
% Param input:
Dinit = Param(1);  %Initial value for Vdc_ref
Dmax = Param(2);   %Maximum value for Vdc_ref
Dmin = Param(3);   %Minimum value for Vdc_ref
deltaD = Param(4); %Increment value used to increase/decrease Vdc_ref
%  

persistent Vold Pold Dold;

dataType = 'double';

if isempty(Vold)
    Vold=0;
    Pold=0;
    Dold=Dinit;
end
P= V*I;
dV= V - Vold;
dP= P - Pold;

if dP ~= 0 & Enabled ~=0
    if dP < 0
        if dV < 0
            D = Dold + deltaD;
        else
            D = Dold - deltaD;
        end
    else
        if dV < 0
            D = Dold - deltaD;
        else
            D = Dold + deltaD;
        end    
    end
else D=Dold;
end

if D >= Dmax | D<= Dmin
    D=Dold;
end

Dold=D;
Vold=V;
Pold=P;
